simulink model "festotemplate_controller"  (R2021b)
settings: Solver=ode45  StartTime=0.0  StopTime=10  RelTol=1e-3  EnableMultiTasking=on
InitFcn:
  | hwinit
values from neighbouring files (symbols this model uses):
  adingain = [1 lasergain  encodergain 1 1 1 1]    [hwinit.m]
  adinoffs = [0 laseroffset encoderoffset 0 0 0 0]    [hwinit.m]
  adoutoff = -0.19    [hwinit.m]
  h = 1e-3    (= 0.001)    [DampingExperiments.m]    (also in FindDamping.m; FindResonance.m; HinfRunFromMatlab.m; Hinfmodel.m)
  K = [-0.3972  -0.8279]    [DampingExperiments.m]    (also in LQGModel.m = place(A,B,[-0.2 + 0.1i -0.2-0.1i]); Model.m = place(A,B,[-0.2 + 0.1i -0.2-0.1i]); RunFromMatlab.m = [-0.3972   -0.8279])
settings Model: Creator=rbabuska  LastModifiedBy=wsboer
settings SolverCC: AlgebraicLoopSolver=TrustRegion
settings DataIOCC: LimitDataPoints=on  SaveFormat=Array  ReturnWorkspaceOutputs=off  SignalLoggingName=sigsOut
settings OptimizationCC: BooleanDataType=off  ExpressionDepthLimit=2147483647  InitFltsAndDblsToZero=on  LifeSpan=inf
settings DebuggingCC: SaveWithParameterizedLinksMsg=none  SignalResolutionControl=TryResolveAllWithWarning  MultiTaskDSMMsg=warning  MultiTaskCondExecSysMsg=none  AllowSymbolicDim=off  StateNameClashWarn=warning  SFUnexpectedBacktrackingDiag=warning  SFNoUnconditionalDefaultTransitionDiag=warning  SFExecutionAtInitializationDiag=none  SFMachineParentedDataDiag=warning  ArithmeticOperatorsInVariantConditions=warning
settings HardwareCC: ProdBitPerPointer=32  ProdBitPerSizeT=32  ProdBitPerPtrDiffT=32  ProdLargestAtomicFloat=None  ProdIntDivRoundTo=Undefined  ProdEndianess=Unspecified  ProdWordSize=32  ProdHWDeviceType=32-bit Generic  TargetUnknown=on
settings ModelReferenceCC: PropagateSignalLabelsOutOfModel=off
settings SFSimCC: SimUseLocalCustomCode=off  CustomCodeUndefinedFunction=UseInterfaceOnly
settings RTWCC: RTWUseLocalCustomCode=off
settings CodeAppCC: StateflowObjectComments=on
settings GRTTargetCC: TargetFcnLib=ansi_tfl_tmw.mat  TargetLangStandard=C89/C90 (ANSI)  CombineOutputUpdateFcns=off  GRTInterface=on
settings ConfigComp: CovMetricSettings=dw  CovSaveCumulativeToWorkspaceVar=on  CovSaveSingleToWorkspaceVar=on  CovExternalEMLEnable=off

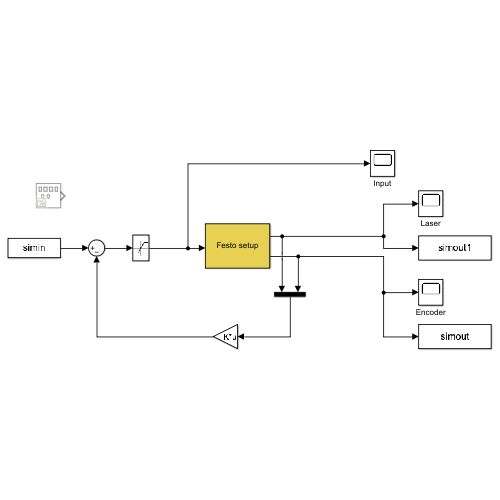
[thumbnail: Simulink's stored preview of the top-level diagram]
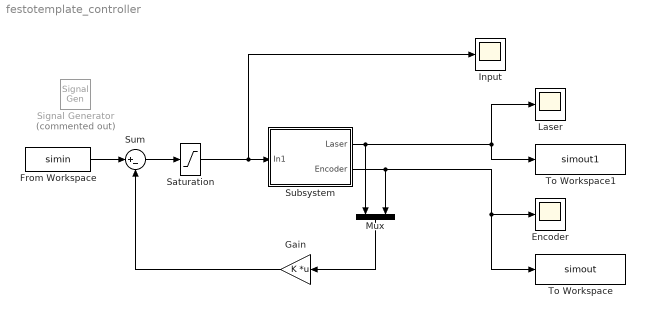
== system festotemplate_controller ==
  Encoder : Scope
  From Workspace : FromWorkspace  VariableName=simin
  Gain : Gain  Gain=K  Multiplication=Matrix(K*u)
  Input : Scope
  Laser : Scope
  Mux : Mux  Inputs=2
  Saturation : Saturate  UpperLimit=5  LowerLimit=-5
  Signal Generator : SignalGenerator  Commented=on  Frequency=14/2.6
  Subsystem : Subsystem
      mask Display: disp('Festo setup')
  Sum : Sum  Inputs=|+-
  To Workspace : ToWorkspace  VariableName=simout  SaveFormat=Timeseries  SampleTime=h
  To Workspace1 : ToWorkspace  VariableName=simout1  SaveFormat=Timeseries  SampleTime=h
  wires:
  Saturation/1 -> Subsystem/1(In1), Input/1
  Subsystem/1(Laser) -> Mux/1, Laser/1, To Workspace1/1
  Subsystem/2(Encoder) -> Mux/2, To Workspace/1, Encoder/1
  Mux/1 -> Gain/1
  Gain/1 -> Sum/2
  From Workspace/1 -> Sum/1
  Sum/1 -> Saturation/1

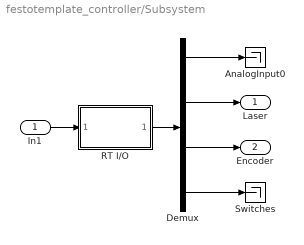
== system festotemplate_controller/Subsystem ==
  In1 : Inport
  AnalogInput0 : Terminator
  Demux : Demux  Outputs=[1 1 1 4]
  RT I/O : Subsystem  mask{Ts=h, channels=[6 7 3]}
      mask prompts: Ts "Sample time [s]:"; channels "The 3 channels to read (e.g. [6 7 3])"
      mask init:
      | hwinit;
      | 
      | % initialize FPGA
      | fugihandle = fugiboard('Open', 'Pendulum1');
      | fugihandle.WatchdogTimeout = 0.5;
      | fugiboard('SetParams', fugihandle);
      | fugiboard('Write', fugihandle, 0, 0, 0, 0);  % dummy write to sync interface board
      | fugiboard('Write', fugihandle, 5, 1, 0, 0);  % reset position, activate relay
      | data = fugiboard('Read', fugihandle);        % get version info from FPGA
      | % model = bitshift(data(1), -5); 
      | % version = bitand(data(1), 31);
      | % disp(sprintf('FPGA setup %d, version %d', model, version)); % for the B&P it should say 1 1, or else there is a problem
      | fugiboard('Write', fugihandle, 0, 1, 0, 0);  % end reset
      | pause(0.1);                         % give relay some time to respond
      mask Display: disp('Flexible\nBeam')
  Switches : Terminator
  Laser : Outport
  Encoder : Outport  Port=2
  wires:
  RT I/O/1(Outputs) -> Demux/1
  In1/1 -> RT I/O/1(Motors)
  Demux/2 -> Laser/1
  Demux/1 -> AnalogInput0/1
  Demux/3 -> Encoder/1
  Demux/4 -> Switches/1

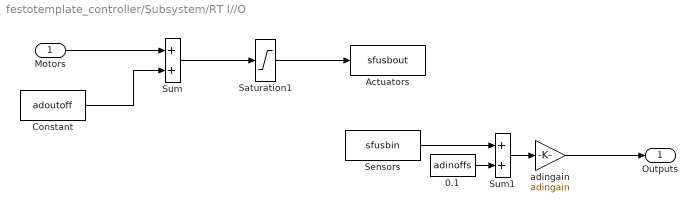
== system festotemplate_controller/Subsystem/RT I//O ==
  Motors : Inport
  0.1 : Constant  Value=adinoffs
  Actuators : S-Function  FunctionName=sfusbout  Parameters=Ts, fugihandle  SFunctionDeploymentMode=off  EnableBusSupport=off
  Constant : Constant  Value=adoutoff
  Saturation1 : Saturate  UpperLimit=10  LowerLimit=-10
  Sensors : S-Function  FunctionName=sfusbin  Parameters=Ts, fugihandle, channels  SFunctionDeploymentMode=off  EnableBusSupport=off
  Sum : Sum  InputSameDT=on  SaturateOnIntegerOverflow=on  OutDataTypeStr=Inherit: Same as first input
  Sum1 : Sum  InputSameDT=on  SaturateOnIntegerOverflow=on  OutDataTypeStr=Inherit: Same as first input
  adingain : Gain  Gain=adingain  SaturateOnIntegerOverflow=on  OutDataTypeStr=Inherit: Same as input  ParamDataTypeStr=Inherit: Same as input
  Outputs : Outport
  wires:
  Motors/1 -> Sum/1
  Sum1/1 -> adingain/1
  0.1/1 -> Sum1/2
  Sensors/1 -> Sum1/1
  adingain/1 -> Outputs/1
  Saturation1/1 -> Actuators/1
  Sum/1 -> Saturation1/1
  Constant/1 -> Sum/2
